simulink model "Expt_3_1"  (R2018a)
settings: Solver=VariableStepAuto  StartTime=0.0  StopTime=10.0  RelTol=1e-3
settings Model: Creator=HP  LastModifiedBy=HP

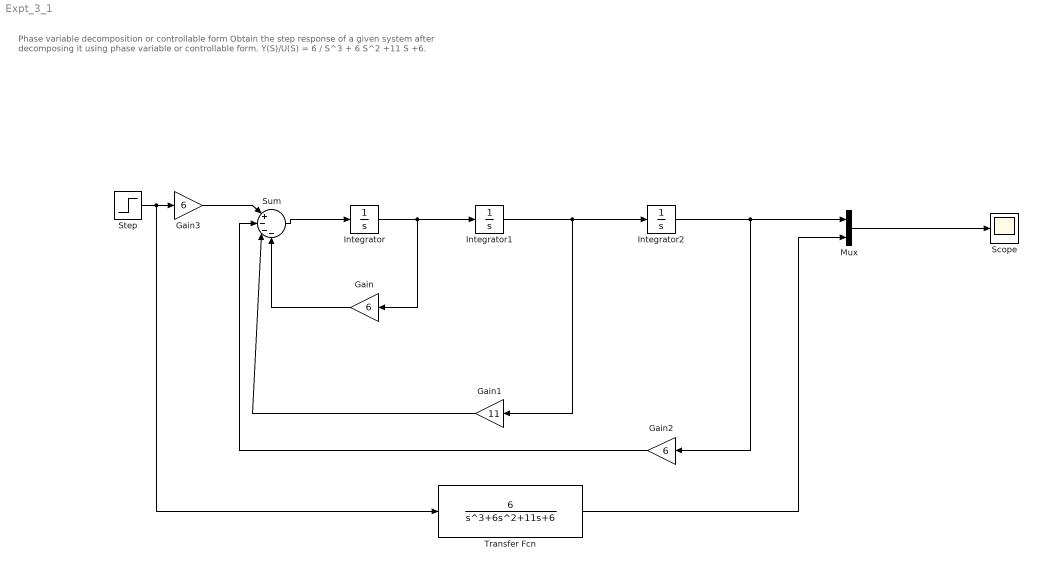
== system Expt_3_1 ==
  note: Phase variable decomposition or controllable form
      |
      | Obtain the step response of a given system after decomposing it using phase variable or controllable form.
      | Y(S)/U(S) = 6 / S^3 + 6 S^2 +11 S +6.
  Gain : Gain  Gain=6
  Gain1 : Gain  Gain=11
  Gain2 : Gain  Gain=6
  Gain3 : Gain  Gain=6
  Integrator : Integrator
  Integrator1 : Integrator
  Integrator2 : Integrator
  Mux : Mux  Inputs=2
  Scope : Scope
  Step : Step  SampleTime=0
  Sum : Sum  Inputs=|+---
  Transfer Fcn : TransferFcn  Numerator=[6]  Denominator=[1 6 11 6]
  wires:
  Integrator2/1 -> Gain2/1, Mux/1
  Integrator1/1 -> Gain1/1, Integrator2/1
  Integrator/1 -> Gain/1, Integrator1/1
  Sum/1 -> Integrator/1
  Step/1 -> Transfer Fcn/1, Gain3/1
  Gain3/1 -> Sum/1
  Gain/1 -> Sum/4
  Gain1/1 -> Sum/3
  Gain2/1 -> Sum/2
  Mux/1 -> Scope/1
  Transfer Fcn/1 -> Mux/2
